simulink model "hw2_sim"  (R2024b)
settings: Solver=VariableStepAuto  StartTime=0.0  StopTime=100  RelTol=1e-3
settings Model: Creator=odm0003  LastModifiedBy=odm0003

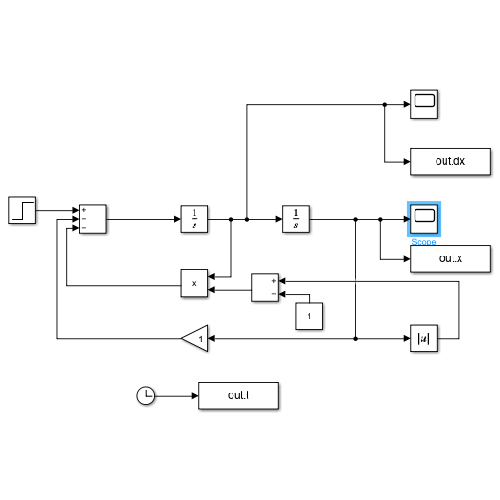
[thumbnail: Simulink's stored preview of the top-level diagram]
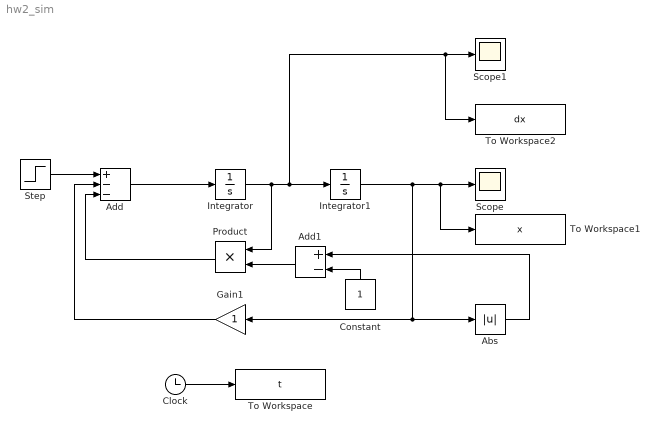
== system hw2_sim ==
  Abs : Abs  SaturateOnIntegerOverflow=off
  Add : Sum  Inputs=+--
  Add1 : Sum  Inputs=+-
  Clock : Clock
  Constant : Constant
  Gain1 : Gain
  Integrator : Integrator
  Integrator1 : Integrator  InitialCondition=5
  Product : Product
  Scope : Scope
  Scope1 : Scope
  Step : Step  After=0  SampleTime=0
  To Workspace : ToWorkspace  VariableName=t  SampleTime=0.1
  To Workspace1 : ToWorkspace  VariableName=x  SampleTime=0.1
  To Workspace2 : ToWorkspace  VariableName=dx  SampleTime=0.1
  wires:
  Step/1 -> Add/1
  Add/1 -> Integrator/1
  Integrator/1 -> Integrator1/1, To Workspace2/1, Scope1/1, Product/1
  Integrator1/1 -> Abs/1, Gain1/1, To Workspace1/1, Scope/1
  Gain1/1 -> Add/2
  Clock/1 -> To Workspace/1
  Add1/1 -> Product/2
  Constant/1 -> Add1/2
  Product/1 -> Add/3
  Abs/1 -> Add1/1
